simulink model "buck"  (R2013a)
settings: Solver=ode23tb  StartTime=0.0  StopTime=10/f  RelTol=1e-4
values from neighbouring files (symbols this model uses):
  C = 220e-6    (= 0.00022)    [boosts.m]
  D = 80    [boosts.m]
  f = 10e3    (= 10000)    [boosts.m]
  L = Lb/2    (= 1.6e-06)    [boosts.m]
  R = 2    [boosts.m]
  V = 12    [boosts.m]
libraries: powerlib_meascontrol x12, powerlib x8
settings Model: Creator=dello  LastModifiedBy=dello
settings SolverCC: SolverResetMethod=Robust
settings DataIOCC: SignalLoggingSaveFormat=ModelDataLogs  SignalLoggingName=results
settings OptimizationCC: BlockReduction=off
settings DebuggingCC: UnconnectedInputMsg=none  UnconnectedOutputMsg=none  UnconnectedLineMsg=none

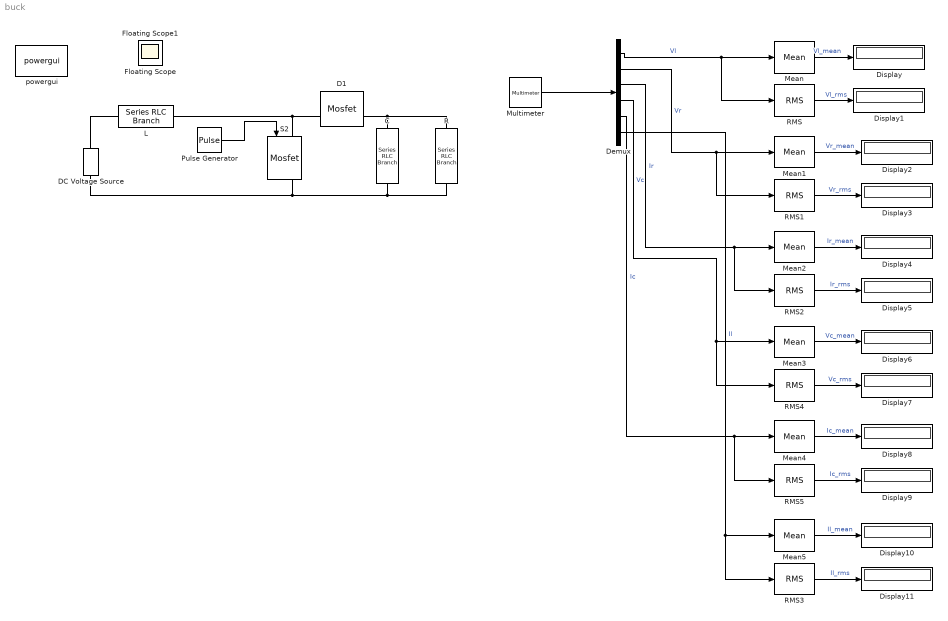
== system buck ==
  C : powerlib/Elements/Series RLC Branch  LConnTagsString=__new0  RConnTagsString=__new0  BranchType=C  Resistance=R  Inductance=1e-3  SetiL0=off  InitialCurrent=0  Capacitance=C  Setx0=off  InitialVoltage=0  Measurements=Branch voltage and current
  D1 : powerlib/Power Electronics/Mosfet  Ron=0.1  Lon=0  Rd=0.01  Vfd=0  IC=0  Rs=1e5  Cs=inf  Measurements=on
  DC Voltage Source : powerlib/Electrical Sources/DC Voltage Source  Amplitude=V  Measurements=None
  Demux : Demux  Outputs=6
  Display{,1..11} (12 alike) : Display
  L : powerlib/Elements/Series RLC Branch  LConnTagsString=__new0  RConnTagsString=__new0  BranchType=L  Resistance=R  Inductance=L  SetiL0=off  InitialCurrent=0  Capacitance=C  Setx0=off  InitialVoltage=0  Measurements=Branch voltage and current
  Mean{,1..5} (6 alike) : powerlib_meascontrol/Measurements/Mean  Freq=f  Vinit=0  Ts=0
  Multimeter : powerlib/Measurements/Multimeter  PhasorSimulation=off  OutputType=Complex  sel=[2 3 6 1 4 5]  L=6  Gain=[1 1 1 1 1 1]  yselected={'Ub: L','Ub: R','Ib: R','Ub: C','Ib: C','Ib: L'};  PSBOutputType=1  PSBequivalent=0  AxesSetting=[0,0.1,-100,100]  Display=0  SavedBlockNames=-11
  Pulse Generator : DiscretePulseGenerator  PulseType=Time based  Period=1/f  PulseWidth=D
  R : powerlib/Elements/Series RLC Branch  LConnTagsString=__new0  RConnTagsString=__new0  BranchType=R  Resistance=R  Inductance=1e-3  SetiL0=off  InitialCurrent=0  Capacitance=1e-6  Setx0=off  InitialVoltage=0  Measurements=Branch voltage and current
  RMS{,1..5} (6 alike) : powerlib_meascontrol/Measurements/RMS  TrueRMS=on  Freq=f  RMSInit=120  Ts=0
  S2 : powerlib/Power Electronics/Mosfet  Ron=0.1  Lon=0  Rd=0.01  Vfd=0  IC=0  Rs=1e5  Cs=inf  Measurements=on
  powergui : powerlib/powergui  Priority=1  SimulationMode=Continuous  SolverType=Tustin  SampleTime=50e-6  frequency=60  SPID=off  DisableSnubberDevices=off  DisableRonSwitches=off  DisableVfSwitches=off  SwTol=0  Interpol=off  DisplayEquations=off  frequencyindice=0  Pbase=100e6  ErrMax=1e-4  Iterations=50  UnitsV=V  UnitsW=W  FunctionMessages=off  echomessages=off  HookPort=off  EnableUseOfTLC=off  x0status=blocks  RestoreLinks=warning  ResistiveCurrentMeasurement=off  Frange=[0:2:500]  Ylog=off  Xlog=on  ShowGrid=off  save=off  variable=ZData  ZoomFFT=off  StartTime=0.0  cycles=1  DisplayStyle=1  fundamental=60  FreqAxis=off  MaxFrequency=1000  frequencyindicesteady=1  RmsSteady=1  display=off  Ts=0  methode=off
  Floating Scope : Scope  NumInputPorts=8
      settings: Floating=on  TimeRange=0.03333333333333333  YMin=-5~-5~-5~-5~-5~-5~-5~-5  YMax=5~5~5~5~5~5~5~5  SaveName=diodes
  Floating Scope1 : Scope
      settings: Floating=on  TimeRange=0.03333333333333333  SaveName=simdata
  wires:
  Multimeter/1 -> Demux/1
  Demux/1 -> RMS/1, Mean/1  "Vl"
  Demux/2 -> RMS1/1, Mean1/1  "Vr"
  Demux/3 -> RMS2/1, Mean2/1  "Ir"
  Mean/1 -> Display/1  "Vl_mean"
  RMS/1 -> Display1/1  "Vl_rms"
  Mean1/1 -> Display2/1  "Vr_mean"
  RMS1/1 -> Display3/1  "Vr_rms"
  Mean2/1 -> Display4/1  "Ir_mean"
  RMS2/1 -> Display5/1  "Ir_rms"
  Demux/4 -> RMS4/1, Mean3/1  "Vc"
  Mean3/1 -> Display6/1  "Vc_mean"
  RMS4/1 -> Display7/1  "Vc_rms"
  Mean4/1 -> Display8/1  "Ic_mean"
  RMS5/1 -> Display9/1  "Ic_rms"
  Demux/5 -> RMS5/1, Mean4/1  "Ic"
  Mean5/1 -> Display10/1  "Il_mean"
  RMS3/1 -> Display11/1  "Il_rms"
  Demux/6 -> RMS3/1, Mean5/1  "Il"
  Pulse Generator/1 -> S2/1
  connections:
  C/RConn1 -- DC Voltage Source/LConn1 -- S2/RConn1 -- R/RConn1
  C/LConn1 -- R/LConn1 -- D1/LConn1
  DC Voltage Source/RConn1 -- L/LConn1
  S2/LConn1 -- D1/RConn1 -- L/RConn1
